simulink model "PDGravityCompensation"  (R2020b)
settings: Solver=VariableStepAuto  StartTime=0.0  StopTime=4  RelTol=1e-3
values from neighbouring files (symbols this model uses):
  Kd = diag([30 40 15])    [params.m]
  Kp = diag([400 380 250])    [params.m]
  qd = [0.3, -0.1, 0.1]    [params.m]
settings Model: Creator=andre  LastModifiedBy=filippo

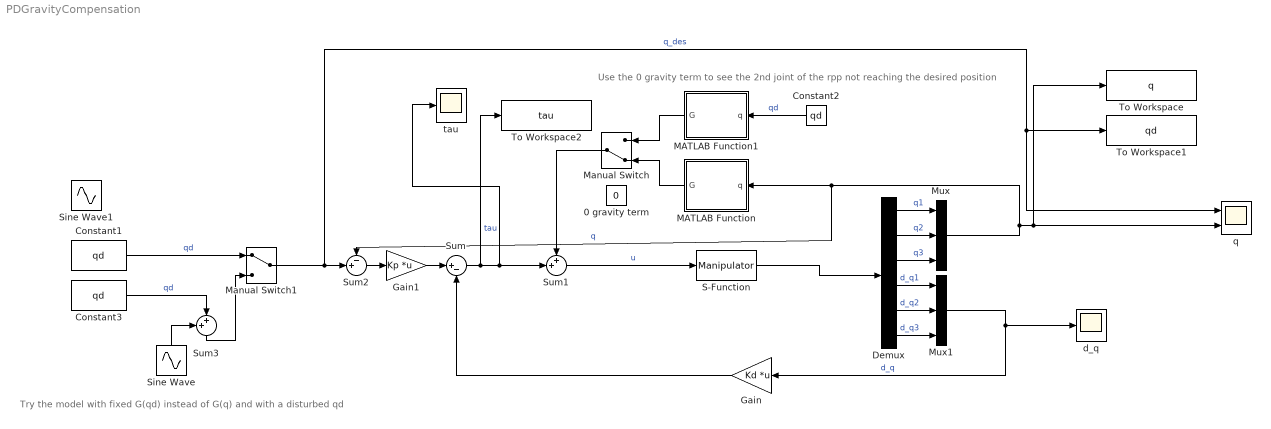
== system PDGravityCompensation ==
  note: Try the model with fixed G(qd) instead of G(q) and with a disturbed qd
  note: Use the 0 gravity term to see the 2nd joint of the rpp not reaching the desired position
  0 gravity term : Constant  Value=0
  Constant1 : Constant  Value=qd
  Constant2 : Constant  Value=qd
  Constant3 : Constant  Value=qd
  Demux : Demux  Outputs=6
  Gain : Gain  Gain=Kd  Multiplication=Matrix(K*u)
  Gain1 : Gain  Gain=Kp  Multiplication=Matrix(K*u)
  MATLAB Function : MATLAB Function  TreatAsAtomicUnit=on
  MATLAB Function1 : MATLAB Function  TreatAsAtomicUnit=on
  Manual Switch : ManualSwitch  CurrentSetting=0
  Manual Switch1 : ManualSwitch
  Mux : Mux  Inputs=3
  Mux1 : Mux  Inputs=3
  S-Function : S-Function  FunctionName=Manipulator  Parameters=param  SFunctionDeploymentMode=off  EnableBusSupport=off
  Sine Wave : Sin  Amplitude=0.01  Frequency=30  SampleTime=0
  Sine Wave1 : Sin  Amplitude=0.1  Frequency=3  SampleTime=0
  Sum : Sum  Inputs=|+-
  Sum1 : Sum  Inputs=++|
  Sum2 : Sum  Inputs=-+|
  Sum3 : Sum  Inputs=++|
  To Workspace : ToWorkspace  VariableName=q  SaveFormat=Timeseries  SampleTime=-1
  To Workspace1 : ToWorkspace  VariableName=qd  SaveFormat=Timeseries  SampleTime=-1
  To Workspace2 : ToWorkspace  VariableName=tau  SaveFormat=Timeseries  SampleTime=-1
  d_q : Scope
  q : Scope  NumInputPorts=2
  tau : Scope
  wires:
  Sum/1 -> tau/1, Sum1/2, To Workspace2/1  "tau"
  Gain1/1 -> Sum/1
  S-Function/1 -> Demux/1
  Demux/3 -> Mux/3  "q3"
  Demux/2 -> Mux/2  "q2"
  Demux/1 -> Mux/1  "q1"
  Demux/4 -> Mux1/1  "d_q1"
  Demux/5 -> Mux1/2  "d_q2"
  Demux/6 -> Mux1/3  "d_q3"
  Mux/1 -> MATLAB Function/1(q), Sum2/1, To Workspace/1, q/2  "q"
  Sum1/1 -> S-Function/1  "u"
  Gain/1 -> Sum/2
  Sum2/1 -> Gain1/1
  Mux1/1 -> d_q/1, Gain/1  "d_q"
  Constant2/1 -> MATLAB Function1/1(q)  "qd"
  MATLAB Function1/1(G) -> Manual Switch/1
  MATLAB Function/1(G) -> Manual Switch/2
  Manual Switch1/1 -> q/1, To Workspace1/1, Sum2/2  "q_des"
  Constant3/1 -> Sum3/2  "qd"
  Sine Wave/1 -> Sum3/1
  Sum3/1 -> Manual Switch1/2
  Constant1/1 -> Manual Switch1/1  "qd"
  Manual Switch/1 -> Sum1/1

== matlab function PDGravityCompensation/MATLAB Function ==
  data: q input; G output; param parameter
function G = Gravity(q, param)
    G = G_Lagrangian(q, param);
end

== matlab function PDGravityCompensation/MATLAB Function1 ==
  data: q input; G output; param parameter
function G = Gravity(q, param)
    G = G_Lagrangian(q, param);
end
